simulink model "SIM1"  (R2023b)
settings: Solver=VariableStepAuto  StartTime=0.0  StopTime=10.0  RelTol=1e-3
libraries: matrix_library x1, vrlib x1
settings Model: Creator=David  LastModifiedBy=David

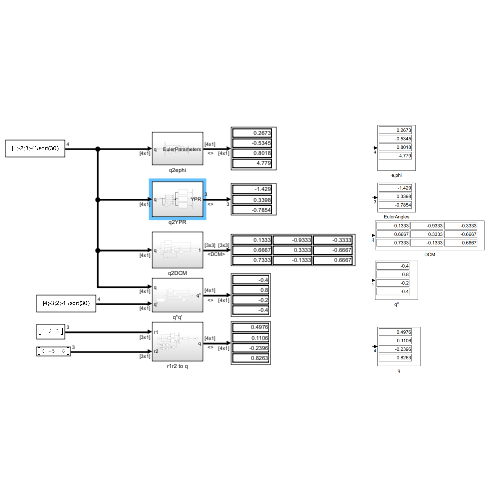
[thumbnail: Simulink's stored preview of the top-level diagram]
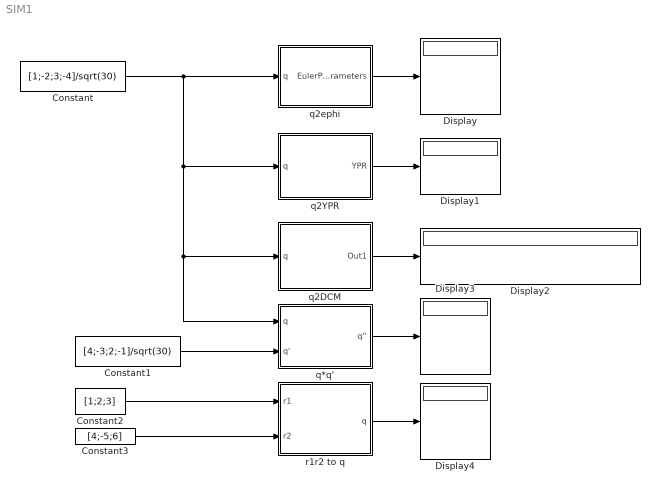
== system SIM1 ==
  Constant : Constant  Value=[1;-2;3;-4]/sqrt(30)
  Constant1 : Constant  Value=[4;-3;2;-1]/sqrt(30)
  Constant2 : Constant  Value=[1;2;3]
  Constant3 : Constant  Value=[4;-5;6]
  Display{,1..4} (5 alike) : Display
  q*q' : Subsystem
  q2DCM : Subsystem
  q2YPR : Subsystem
  q2ephi : Subsystem
  r1r2 to q : Subsystem
  wires:
  Constant/1 -> q*q'/1(q), q2DCM/1(q), q2YPR/1(q), q2ephi/1(q)
  Constant2/1 -> r1r2 to q/1(r1)
  Constant3/1 -> r1r2 to q/2(r2)
  Constant1/1 -> q*q'/2(q')
  q2ephi/1(EulerParameters) -> Display/1
  q2YPR/1(YPR) -> Display1/1
  q2DCM/1(Out1) -> Display2/1
  q*q'/1(q'') -> Display3/1
  r1r2 to q/1(q) -> Display4/1

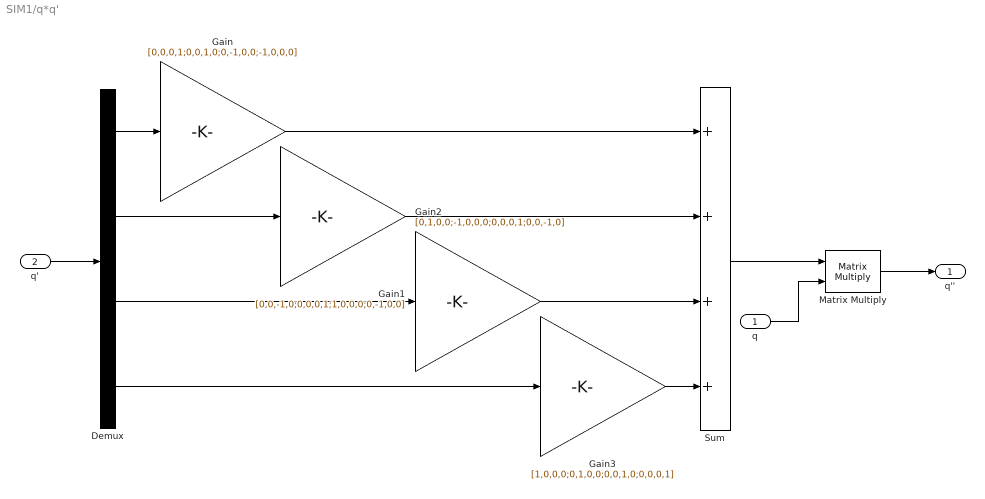
== system SIM1/q*q' ==
  q : Inport  PortDimensions=[4,1]
  q' : Inport  Port=2  PortDimensions=[4,1]
  Demux : Demux
  Gain : Gain  Gain=[0,0,0,1;0,0,1,0;0,-1,0,0;-1,0,0,0]
  Gain1 : Gain  Gain=[0,0,-1,0;0,0,0,1;1,0,0,0;0,-1,0,0]
  Gain2 : Gain  Gain=[0,1,0,0;-1,0,0,0;0,0,0,1;0,0,-1,0]
  Gain3 : Gain  Gain=[1,0,0,0;0,1,0,0;0,0,1,0;0,0,0,1]
  Matrix Multiply : Product  Multiplication=Matrix(*)
  Sum : Sum  Inputs=++++
  q'' : Outport
  wires:
  q'/1 -> Demux/1
  Demux/1 -> Gain/1
  Demux/2 -> Gain1/1
  Demux/4 -> Gain3/1
  Demux/3 -> Gain2/1
  Gain2/1 -> Sum/3
  Gain3/1 -> Sum/4
  Gain1/1 -> Sum/2
  Gain/1 -> Sum/1
  Sum/1 -> Matrix Multiply/1
  q/1 -> Matrix Multiply/2
  Matrix Multiply/1 -> q''/1

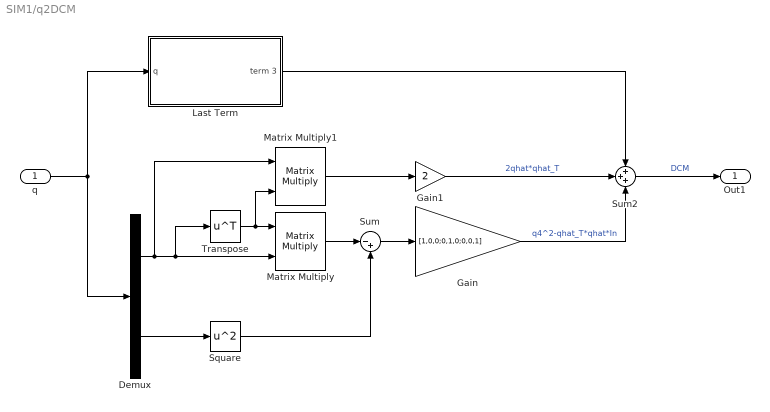
== system SIM1/q2DCM ==
  q : Inport  PortDimensions=[4,1]
  Demux : Demux  Outputs=[3,1]
  Gain : Gain  Gain=[1,0,0;0,1,0;0,0,1]
  Gain1 : Gain  Gain=2
  Last Term : Subsystem
  Matrix Multiply : Product  Multiplication=Matrix(*)
  Matrix Multiply1 : Product  Multiplication=Matrix(*)
  Square : Math  Operator=square
  Sum : Sum  Inputs=|-+
  Sum2 : Sum  Inputs=+++
  Transpose : Math  Operator=transpose
  Out1 : Outport
  wires:
  Demux/2 -> Square/1
  Demux/1 -> Matrix Multiply1/1, Transpose/1, Matrix Multiply/2
  Transpose/1 -> Matrix Multiply1/2, Matrix Multiply/1
  Matrix Multiply/1 -> Sum/1
  Square/1 -> Sum/2
  Sum/1 -> Gain/1
  q/1 -> Last Term/1(q), Demux/1
  Matrix Multiply1/1 -> Gain1/1
  Sum2/1 -> Out1/1  "DCM"
  Gain1/1 -> Sum2/2  "2qhat*qhat_T"
  Gain/1 -> Sum2/3  "q4^2-qhat_T*qhat*In"
  Last Term/1(term 3) -> Sum2/1

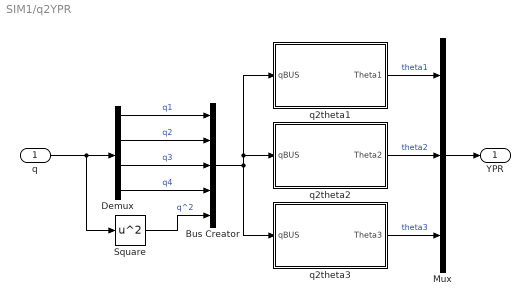
== system SIM1/q2YPR ==
  q : Inport  PortDimensions=[4,1]
  Bus Creator : BusCreator  Inputs=5
  Demux : Demux
  Mux : Mux  Inputs=3
  Square : Math  Operator=square
  q2theta1 : Subsystem
  q2theta2 : Subsystem
  q2theta3 : Subsystem
  YPR : Outport
  wires:
  q/1 -> Square/1, Demux/1
  Demux/1 -> Bus Creator/1  "q1"
  Demux/2 -> Bus Creator/2  "q2"
  Demux/3 -> Bus Creator/3  "q3"
  Demux/4 -> Bus Creator/4  "q4"
  Bus Creator/1 -> q2theta3/1(qBUS), q2theta1/1(qBUS), q2theta2/1(qBUS)
  q2theta1/1(Theta1) -> Mux/1  "theta1"
  q2theta2/1(Theta2) -> Mux/2  "theta2"
  q2theta3/1(Theta3) -> Mux/3  "theta3"
  Mux/1 -> YPR/1
  Square/1 -> Bus Creator/5  "q^2"

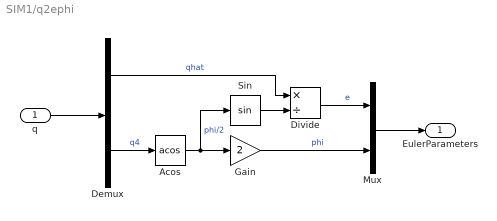
== system SIM1/q2ephi ==
  q : Inport  PortDimensions=[4;1]
  Acos : Trigonometry  Operator=acos
  Demux : Demux  Outputs=[3,1]
  Divide : Product  Inputs=*/
  Gain : Gain  Gain=2
  Mux : Mux  Inputs=2
  Sin : Trigonometry
  EulerParameters : Outport
  wires:
  q/1 -> Demux/1
  Acos/1 -> Gain/1, Sin/1  "phi/2"
  Sin/1 -> Divide/2
  Demux/1 -> Divide/1  "qhat"
  Demux/2 -> Acos/1  "q4"
  Divide/1 -> Mux/1  "e"
  Gain/1 -> Mux/2  "phi"
  Mux/1 -> EulerParameters/1

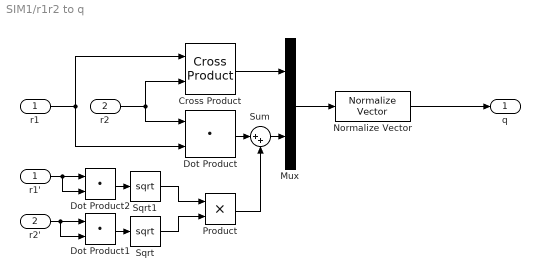
== system SIM1/r1r2 to q ==
  r1 : Inport  PortDimensions=[3;1]
  r2 : Inport  Port=2  PortDimensions=[3;1]
  Cross Product : matrix_library/Cross Product
  Dot Product : DotProduct  OutDataTypeStr=Inherit: Inherit via internal rule
  Dot Product1 : DotProduct  OutDataTypeStr=Inherit: Inherit via internal rule
  Dot Product2 : DotProduct  OutDataTypeStr=Inherit: Inherit via internal rule
  Mux : Mux  Inputs=2
  Normalize Vector : vrlib/Utilities/Normalize Vector  maxzero=0
  Product : Product
  Sqrt : Sqrt
  Sqrt1 : Sqrt
  Sum : Sum  Inputs=|++
  r1' : InportShadow  PortDimensions=[3;1]
  r2' : InportShadow  Port=2  PortDimensions=[3;1]
  q : Outport
  wires:
  r1/1 -> Cross Product/1, Dot Product/2
  r2/1 -> Dot Product/1, Cross Product/2
  Cross Product/1 -> Mux/1
  Mux/1 -> Normalize Vector/1
  Normalize Vector/1 -> q/1
  Dot Product/1 -> Sum/1
  Sum/1 -> Mux/2
  r2'/1 -> Dot Product1/2, Dot Product1/1
  Dot Product1/1 -> Sqrt/1
  Product/1 -> Sum/2
  Dot Product2/1 -> Sqrt1/1
  r1'/1 -> Dot Product2/2, Dot Product2/1
  Sqrt1/1 -> Product/1
  Sqrt/1 -> Product/2

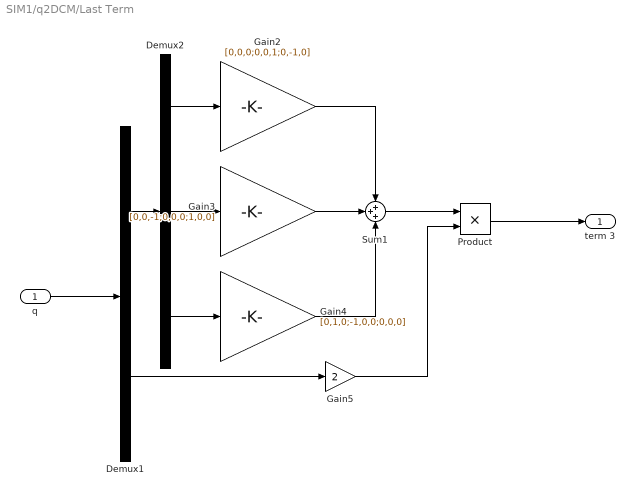
== system SIM1/q2DCM/Last Term ==
  q : Inport
  Demux1 : Demux  Outputs=[3,1]
  Demux2 : Demux  Outputs=3
  Gain2 : Gain  Gain=[0,0,0;0,0,1;0,-1,0]
  Gain3 : Gain  Gain=[0,0,-1;0,0,0;1,0,0]
  Gain4 : Gain  Gain=[0,1,0;-1,0,0;0,0,0]
  Gain5 : Gain  Gain=2
  Product : Product
  Sum1 : Sum  Inputs=+++
  term 3 : Outport
  wires:
  Gain4/1 -> Sum1/3
  Demux2/3 -> Gain4/1
  Demux2/2 -> Gain3/1
  Demux1/2 -> Gain5/1
  Sum1/1 -> Product/1
  Gain2/1 -> Sum1/1
  Demux2/1 -> Gain2/1
  Gain3/1 -> Sum1/2
  Gain5/1 -> Product/2
  Demux1/1 -> Demux2/1
  Product/1 -> term 3/1
  q/1 -> Demux1/1

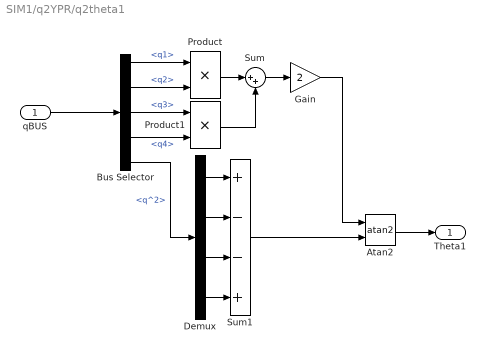
== system SIM1/q2YPR/q2theta1 ==
  qBUS : Inport
  Atan2 : Trigonometry  Operator=atan2
  Bus Selector : BusSelector  OutputSignals=q1,q2,q3,q4,q^2
  Demux : Demux
  Gain : Gain  Gain=2
  Product : Product
  Product1 : Product
  Sum : Sum  Inputs=|++
  Sum1 : Sum  Inputs=+--+
  Theta1 : Outport
  wires:
  qBUS/1 -> Bus Selector/1
  Atan2/1 -> Theta1/1
  Bus Selector/1 -> Product/1  "<q1>"
  Bus Selector/2 -> Product/2  "<q2>"
  Bus Selector/3 -> Product1/1  "<q3>"
  Bus Selector/4 -> Product1/2  "<q4>"
  Product/1 -> Sum/1
  Product1/1 -> Sum/2
  Sum/1 -> Gain/1
  Gain/1 -> Atan2/1
  Demux/1 -> Sum1/1
  Demux/2 -> Sum1/2
  Demux/3 -> Sum1/3
  Demux/4 -> Sum1/4
  Sum1/1 -> Atan2/2
  Bus Selector/5 -> Demux/1  "<q^2>"

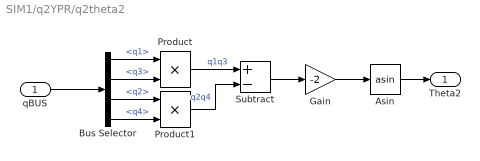
== system SIM1/q2YPR/q2theta2 ==
  qBUS : Inport
  Asin : Trigonometry  Operator=asin
  Bus Selector : BusSelector  OutputSignals=q1,q3,q2,q4
  Gain : Gain  Gain=-2
  Product : Product
  Product1 : Product
  Subtract : Sum  Inputs=+-
  Theta2 : Outport
  wires:
  qBUS/1 -> Bus Selector/1
  Bus Selector/1 -> Product/1  "<q1>"
  Bus Selector/2 -> Product/2  "<q3>"
  Bus Selector/3 -> Product1/1  "<q2>"
  Bus Selector/4 -> Product1/2  "<q4>"
  Product/1 -> Subtract/1  "q1q3"
  Product1/1 -> Subtract/2  "q2q4"
  Subtract/1 -> Gain/1
  Gain/1 -> Asin/1
  Asin/1 -> Theta2/1

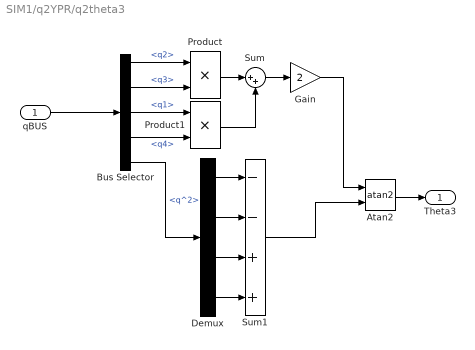
== system SIM1/q2YPR/q2theta3 ==
  qBUS : Inport
  Atan2 : Trigonometry  Operator=atan2
  Bus Selector : BusSelector  OutputSignals=q2,q3,q1,q4,q^2
  Demux : Demux
  Gain : Gain  Gain=2
  Product : Product
  Product1 : Product
  Sum : Sum  Inputs=|++
  Sum1 : Sum  Inputs=--++
  Theta3 : Outport
  wires:
  qBUS/1 -> Bus Selector/1
  Atan2/1 -> Theta3/1
  Product/1 -> Sum/1
  Product1/1 -> Sum/2
  Sum/1 -> Gain/1
  Gain/1 -> Atan2/1
  Demux/1 -> Sum1/1
  Demux/2 -> Sum1/2
  Demux/3 -> Sum1/3
  Demux/4 -> Sum1/4
  Sum1/1 -> Atan2/2
  Bus Selector/1 -> Product/1  "<q2>"
  Bus Selector/2 -> Product/2  "<q3>"
  Bus Selector/3 -> Product1/1  "<q1>"
  Bus Selector/4 -> Product1/2  "<q4>"
  Bus Selector/5 -> Demux/1  "<q^2>"
